simulink library "INT_CrCtl_StM"  (R2016b)
settings: Solver=VariableStepAuto  StartTime=0.0  StopTime=10.0  RelTol=1e-3
settings Model: Creator=guanxiaoxing  LastModifiedBy=guanxiaoxing

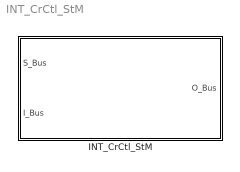
== system INT_CrCtl_StM ==
  INT_CrCtl_StM : Subsystem

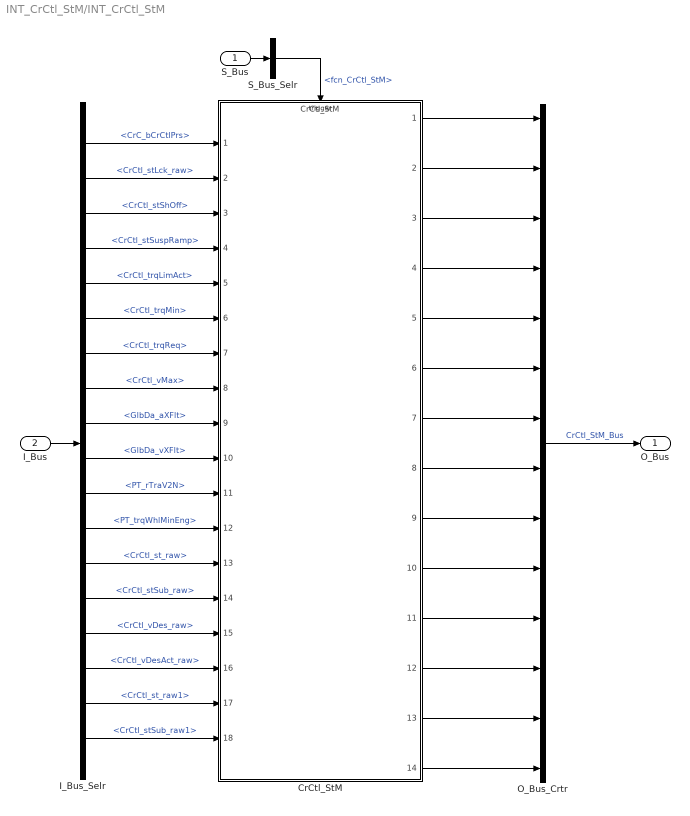
== system INT_CrCtl_StM/INT_CrCtl_StM ==
  S_Bus : Inport
  I_Bus : Inport  Port=2
  CrCtl_StM : ModelReference  ModelNameDialog=CrCtl_StM  SimulationMode=Normal  ModelReferenceVersion=1.78  TriggerPortName=function  TriggerPortTriggerType=function-call  TriggerPortStatesWhenEnabling=held
  I_Bus_Selr : BusSelector  OutputSignals=CrC_bCrCtlPrs,CrCtl_stLck_raw,CrCtl_stShOff,CrCtl_stSuspRamp,CrCtl_trqLimAct,CrCtl_trqMin,CrCtl_trqReq,CrCtl_vMax,GlbDa_aXFlt,GlbDa_vXFlt,PT_rTraV2N,PT_trqWhlMinEng,CrCtl_st_raw,CrCtl_stSub_raw,CrCtl_vDes_raw,CrCtl_vDesAct_raw,CrCtl_st_raw1,CrCtl_stSub_raw1
  O_Bus_Crtr : BusCreator  Inputs=14
  S_Bus_Selr : BusSelector  OutputSignals=fcn_CrCtl_StM
  O_Bus : Outport
  wires:
  S_Bus_Selr/1 -> CrCtl_StM/Trigger  "<fcn_CrCtl_StM>"
  S_Bus/1 -> S_Bus_Selr/1
  I_Bus/1 -> I_Bus_Selr/1
  I_Bus_Selr/1 -> CrCtl_StM/1  "<CrC_bCrCtlPrs>"
  I_Bus_Selr/2 -> CrCtl_StM/2  "<CrCtl_stLck_raw>"
  I_Bus_Selr/3 -> CrCtl_StM/3  "<CrCtl_stShOff>"
  I_Bus_Selr/4 -> CrCtl_StM/4  "<CrCtl_stSuspRamp>"
  I_Bus_Selr/5 -> CrCtl_StM/5  "<CrCtl_trqLimAct>"
  I_Bus_Selr/6 -> CrCtl_StM/6  "<CrCtl_trqMin>"
  I_Bus_Selr/7 -> CrCtl_StM/7  "<CrCtl_trqReq>"
  I_Bus_Selr/8 -> CrCtl_StM/8  "<CrCtl_vMax>"
  I_Bus_Selr/9 -> CrCtl_StM/9  "<GlbDa_aXFlt>"
  I_Bus_Selr/10 -> CrCtl_StM/10  "<GlbDa_vXFlt>"
  I_Bus_Selr/11 -> CrCtl_StM/11  "<PT_rTraV2N>"
  I_Bus_Selr/12 -> CrCtl_StM/12  "<PT_trqWhlMinEng>"
  I_Bus_Selr/13 -> CrCtl_StM/13  "<CrCtl_st_raw>"
  I_Bus_Selr/14 -> CrCtl_StM/14  "<CrCtl_stSub_raw>"
  I_Bus_Selr/15 -> CrCtl_StM/15  "<CrCtl_vDes_raw>"
  I_Bus_Selr/16 -> CrCtl_StM/16  "<CrCtl_vDesAct_raw>"
  I_Bus_Selr/17 -> CrCtl_StM/17  "<CrCtl_st_raw1>"
  I_Bus_Selr/18 -> CrCtl_StM/18  "<CrCtl_stSub_raw1>"
  O_Bus_Crtr/1 -> O_Bus/1  "CrCtl_StM_Bus"
  CrCtl_StM/1 -> O_Bus_Crtr/1
  CrCtl_StM/2 -> O_Bus_Crtr/2
  CrCtl_StM/3 -> O_Bus_Crtr/3
  CrCtl_StM/4 -> O_Bus_Crtr/4
  CrCtl_StM/5 -> O_Bus_Crtr/5
  CrCtl_StM/6 -> O_Bus_Crtr/6
  CrCtl_StM/7 -> O_Bus_Crtr/7
  CrCtl_StM/8 -> O_Bus_Crtr/8
  CrCtl_StM/9 -> O_Bus_Crtr/9
  CrCtl_StM/10 -> O_Bus_Crtr/10
  CrCtl_StM/11 -> O_Bus_Crtr/11
  CrCtl_StM/12 -> O_Bus_Crtr/12
  CrCtl_StM/13 -> O_Bus_Crtr/13
  CrCtl_StM/14 -> O_Bus_Crtr/14
